simulink model "SL7_2_151_org"  (Simulink 10.0)
settings: Solver=VariableStepAuto  StartTime=0.0  StopTime=10.0  RelTol=1e-3  EnableMultiTasking=on
libraries: simulink x1
settings Model: Creator=Administrator  LastModifiedBy=bhisma
settings DataIOCC: LimitDataPoints=on  SaveFormat=Dataset
settings DebuggingCC: UnderspecifiedInitializationDetection=Simplified  MergeDetectMultiDrivingBlocksExec=error  AllowSymbolicDim=off
settings HardwareCC: ProdBitPerPointer=64  ProdBitPerSizeT=64  ProdBitPerPtrDiffT=64  ProdLargestAtomicFloat=Float  ProdIntDivRoundTo=Zero  ProdEndianess=LittleEndian  ProdWordSize=64  ProdHWDeviceType=Intel->x86-64 (Windows64)
settings GRTTargetCC: CombineOutputUpdateFcns=on  GRTInterface=off
settings ConfigComp: CovExternalEMLEnable=off

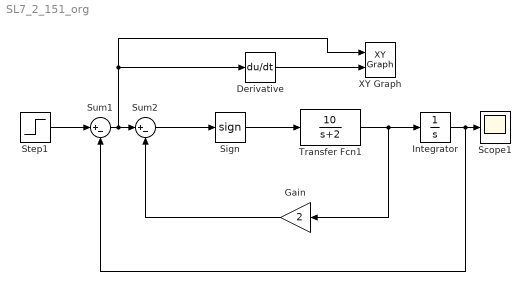
== system SL7_2_151_org ==
  Derivative : Derivative
  Gain : Gain  Gain=2
  Integrator : Integrator
  Scope1 : Scope
  Sign : Signum  ZeroCross=off
  Step1 : Step  Time=0  SampleTime=0
  Sum1 : Sum  Inputs=|+-
  Sum2 : Sum  Inputs=|+-
  Transfer Fcn1 : TransferFcn  Numerator=[10]  Denominator=[1 2]
  XY Graph : simulink/Sinks/XY Graph  xmin=0.7  xmax=1.2  ymin=-1  ymax=1  st=-1
  wires:
  Transfer Fcn1/1 -> Gain/1, Integrator/1
  Step1/1 -> Sum1/1
  Sum1/1 -> Sum2/1, Derivative/1, XY Graph/1
  Gain/1 -> Sum2/2
  Integrator/1 -> Sum1/2, Scope1/1
  Derivative/1 -> XY Graph/2
  Sign/1 -> Transfer Fcn1/1
  Sum2/1 -> Sign/1
